simulink model "ProjectSimulation"  (R2024b)
settings: Solver=ode45  StartTime=0.0  StopTime=5.0  MaxStep=0.001  RelTol=1e-6  AbsTol=1e-6
settings Model: Creator=erens  LastModifiedBy=erens
settings DataIOCC: SaveOutput=off  SignalLogging=off  DSMLogging=off  SaveTime=off  ReturnWorkspaceOutputs=off

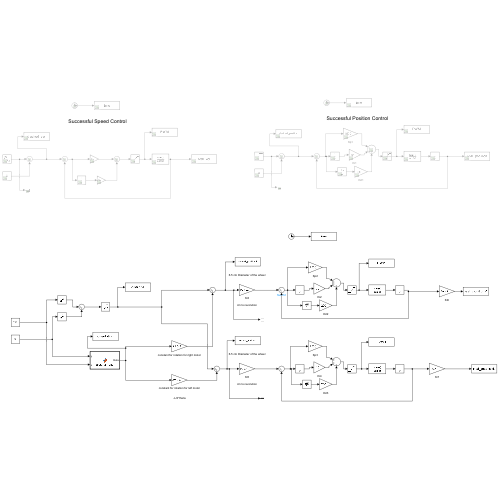
[thumbnail: Simulink's stored preview of the top-level diagram]
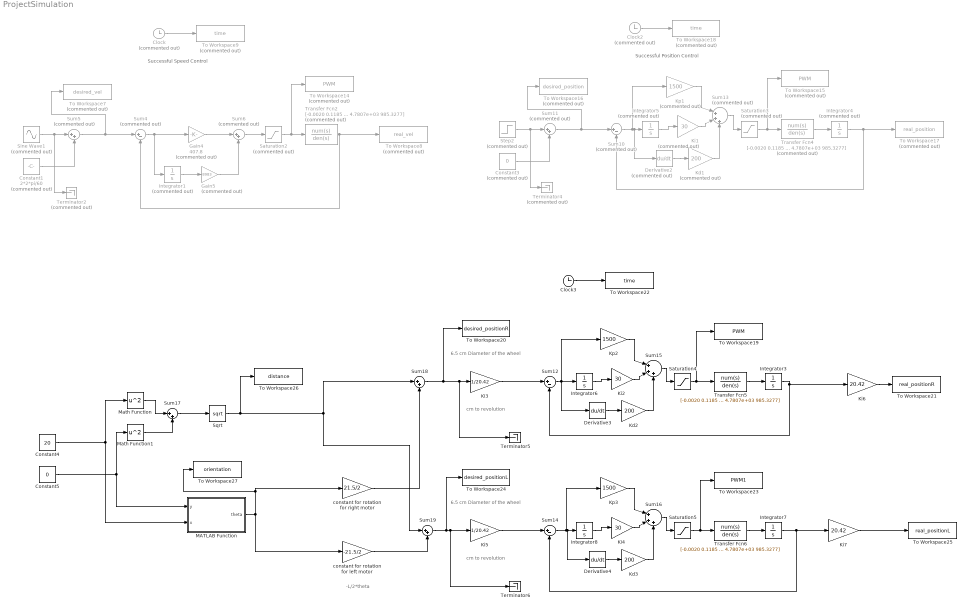
== system ProjectSimulation ==
  note: 6.5 cm Diameter of the wheel
  note: cm to revolution
  note: cm to revolution
  note: 6.5 cm Diameter of the wheel
  note: Successful Position Control
  note: Successful Speed Control
  note: -L/2*theta
  Clock : Clock  Commented=on
  Clock2 : Clock  Commented=on
  Clock3 : Clock
  Constant1 : Constant  Commented=on  Value=2*2*pi/60
  Constant3 : Constant  Commented=on  Value=0
  Constant4 : Constant  Value=20
  Constant5 : Constant  Value=0
  Derivative2 : Derivative  Commented=on
  Derivative3 : Derivative
  Derivative4 : Derivative
  Gain4 : Gain  Commented=on  Gain=407.8
  Gain5 : Gain  Commented=on  Gain=8983
  Integrator1 : Integrator  Commented=on
  Integrator{3,6..8} (4 alike) : Integrator
  Integrator4 : Integrator  Commented=on
  Integrator5 : Integrator  Commented=on
  Kd1 : Gain  Commented=on  Gain=200
  Kd2 : Gain  Gain=200
  Kd3 : Gain  Gain=200
  Ki1 : Gain  Commented=on  Gain=30
  Ki2 : Gain  Gain=30
  Ki3 : Gain  Gain=1/20.42
  Ki4 : Gain  Gain=30
  Ki5 : Gain  Gain=1/20.42
  Ki6 : Gain  Gain=20.42
  Ki7 : Gain  Gain=20.42
  Kp1 : Gain  Commented=on  Gain=1500
  Kp2 : Gain  Gain=1500
  Kp3 : Gain  Gain=1500
  MATLAB Function : MATLAB Function  TreatAsAtomicUnit=on
  Math Function : Math  Operator=square
  Math Function1 : Math  Operator=square
  Saturation2 : Saturate  Commented=on  UpperLimit=255  LowerLimit=0
  Saturation3 : Saturate  Commented=on  UpperLimit=255  LowerLimit=0
  Saturation4 : Saturate  UpperLimit=255  LowerLimit=0
  Saturation5 : Saturate  UpperLimit=255  LowerLimit=0
  Sine Wave1 : Sin  Commented=on  Amplitude=2*2*pi/60  Frequency=1*pi*2  SampleTime=0
  Sqrt : Sqrt
  Step2 : Step  Commented=on  SampleTime=0
  Sum10 : Sum  Commented=on  Inputs=|+-
  Sum11 : Sum  Commented=on  Inputs=|++
  Sum12 : Sum  Inputs=|+-
  Sum13 : Sum  Commented=on  Inputs=|+++
  Sum14 : Sum  Inputs=|+-
  Sum15 : Sum  Inputs=|+++
  Sum16 : Sum  Inputs=|+++
  Sum17 : Sum  Inputs=|++
  Sum18 : Sum  Inputs=|++
  Sum19 : Sum  Inputs=|++
  Sum4 : Sum  Commented=on  Inputs=|+-
  Sum5 : Sum  Commented=on  Inputs=|++
  Sum6 : Sum  Commented=on  Inputs=|++
  Terminator2 : Terminator  Commented=on
  Terminator4 : Terminator  Commented=on
  Terminator5 : Terminator
  Terminator6 : Terminator
  To Workspace14 : ToWorkspace  Commented=on  VariableName=PWM  SampleTime=-1
  To Workspace15 : ToWorkspace  Commented=on  VariableName=PWM  SampleTime=-1
  To Workspace16 : ToWorkspace  Commented=on  VariableName=desired_position  SampleTime=-1
  To Workspace17 : ToWorkspace  Commented=on  VariableName=real_position  SampleTime=-1
  To Workspace18 : ToWorkspace  Commented=on  VariableName=time  SampleTime=-1
  To Workspace19 : ToWorkspace  VariableName=PWM  SampleTime=-1
  To Workspace20 : ToWorkspace  VariableName=desired_positionR  SampleTime=-1
  To Workspace21 : ToWorkspace  VariableName=real_positionR  SampleTime=-1
  To Workspace22 : ToWorkspace  VariableName=time  SampleTime=-1
  To Workspace23 : ToWorkspace  VariableName=PWM1  SampleTime=-1
  To Workspace24 : ToWorkspace  VariableName=desired_positionL  SampleTime=-1
  To Workspace25 : ToWorkspace  VariableName=real_positionL  SampleTime=-1
  To Workspace26 : ToWorkspace  VariableName=distance  SampleTime=-1
  To Workspace27 : ToWorkspace  VariableName=orientation  SampleTime=-1
  To Workspace7 : ToWorkspace  Commented=on  VariableName=desired_vel  SampleTime=-1
  To Workspace8 : ToWorkspace  Commented=on  VariableName=real_vel  SampleTime=-1
  To Workspace9 : ToWorkspace  Commented=on  VariableName=time  SampleTime=-1
  Transfer Fcn2 : TransferFcn  Commented=on  Numerator=[-0.0020 0.1185 1.5838 32.4776 6.3667]  Denominator=[1 26.9721 822.6898 4.7807e+03 985.3277]
  Transfer Fcn4 : TransferFcn  Commented=on  Numerator=[-0.0020 0.1185 1.5838 32.4776 6.3667]  Denominator=[1 26.9721 822.6898 4.7807e+03 985.3277]
  Transfer Fcn5 : TransferFcn  Numerator=[-0.0020 0.1185 1.5838 32.4776 6.3667]  Denominator=[1 26.9721 822.6898 4.7807e+03 985.3277]
  Transfer Fcn6 : TransferFcn  Numerator=[-0.0020 0.1185 1.5838 32.4776 6.3667]  Denominator=[1 26.9721 822.6898 4.7807e+03 985.3277]
  constant for rotation for left motor : Gain  Gain=-21.5/2
  constant for rotation for right motor : Gain  Gain=21.5/2
  wires:
  Sum4/1 -> Integrator1/1, Gain4/1
  Integrator1/1 -> Gain5/1
  Constant1/1 -> Sum5/2
  Sum5/1 -> Sum4/1, To Workspace7/1
  Gain4/1 -> Sum6/1
  Transfer Fcn2/1 -> Sum4/2, To Workspace8/1
  Sine Wave1/1 -> Terminator2/1, Sum5/1
  Gain5/1 -> Sum6/2
  Clock/1 -> To Workspace9/1
  Sum6/1 -> Saturation2/1
  Saturation2/1 -> To Workspace14/1, Transfer Fcn2/1
  Saturation3/1 -> To Workspace15/1, Transfer Fcn4/1
  Constant3/1 -> Sum11/2
  Step2/1 -> Terminator4/1, Sum11/1
  Sum11/1 -> Sum10/1, To Workspace16/1
  Clock2/1 -> To Workspace18/1
  Transfer Fcn4/1 -> Integrator4/1
  Integrator4/1 -> Sum10/2, To Workspace17/1
  Kp1/1 -> Sum13/1
  Integrator5/1 -> Ki1/1
  Ki1/1 -> Sum13/2
  Derivative2/1 -> Kd1/1
  Sum10/1 -> Kp1/1, Derivative2/1, Integrator5/1
  Kd1/1 -> Sum13/3
  Sum13/1 -> Saturation3/1
  Sum12/1 -> Derivative3/1, Integrator6/1, Kp2/1
  Ki2/1 -> Sum15/2
  Integrator6/1 -> Ki2/1
  Derivative3/1 -> Kd2/1
  Kp2/1 -> Sum15/1
  Ki3/1 -> Sum12/1
  Integrator3/1 -> Ki6/1, Sum12/2
  Sum15/1 -> Saturation4/1
  Saturation4/1 -> To Workspace19/1, Transfer Fcn5/1
  Clock3/1 -> To Workspace22/1
  Transfer Fcn5/1 -> Integrator3/1
  Kd2/1 -> Sum15/3
  Sum18/1 -> Terminator5/1, Ki3/1, To Workspace20/1
  Ki5/1 -> Sum14/1
  Transfer Fcn6/1 -> Integrator7/1
  Kd3/1 -> Sum16/3
  Saturation5/1 -> To Workspace23/1, Transfer Fcn6/1
  Integrator7/1 -> Ki7/1, Sum14/2
  Sum16/1 -> Saturation5/1
  Derivative4/1 -> Kd3/1
  Kp3/1 -> Sum16/1
  Sum19/1 -> Terminator6/1, Ki5/1, To Workspace24/1
  Integrator8/1 -> Ki4/1
  Ki4/1 -> Sum16/2
  Sum14/1 -> Kp3/1, Derivative4/1, Integrator8/1
  Constant4/1 -> MATLAB Function/2(x), Math Function/1
  Constant5/1 -> Math Function1/1, MATLAB Function/1(y)
  Math Function/1 -> Sum17/1
  Math Function1/1 -> Sum17/2
  Sum17/1 -> Sqrt/1
  Sqrt/1 -> Sum19/1, Sum18/1, To Workspace26/1
  MATLAB Function/1(theta) -> constant for rotation for right motor/1, To Workspace27/1, constant for rotation for left motor/1
  constant for rotation for right motor/1 -> Sum18/2
  constant for rotation for left motor/1 -> Sum19/2
  Ki6/1 -> To Workspace21/1
  Ki7/1 -> To Workspace25/1

== matlab function ProjectSimulation/MATLAB Function ==
  data: y input; theta output; x input
function theta = arctan2_func(y, x)
%#codegen
    theta = atan2(y, x);
end
